simulink subsystem "ElectricMachine1"  (R2022b)
settings: Solver=VariableStepAuto  StartTime=0.0  StopTime=10.0  RelTol=1e-3
undefined symbols (not defined in the file): Spark_MaxTrq_Spd, Spark_Spd_BrkPts
libraries: autolibmappedmotor x1
settings Model: ModifiedByFormat=The MathWorks, Inc.  Creator=The MathWorks, Inc.  LastModifiedBy=The MathWorks, Inc.
settings SolverCC: MaxZcPerStep=1
settings DebuggingCC: UnconnectedInputMsg=warning  UnconnectedOutputMsg=warning  UnconnectedLineMsg=warning
settings ModelReferenceCC: EnableRefExpFcnMdlSchedulingChecks=on
settings RTWCC: DLArmComputeVersion=19.05

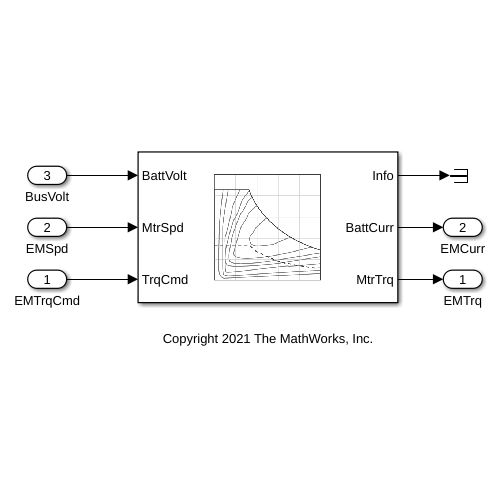
[thumbnail: Simulink's stored preview of the top-level diagram]
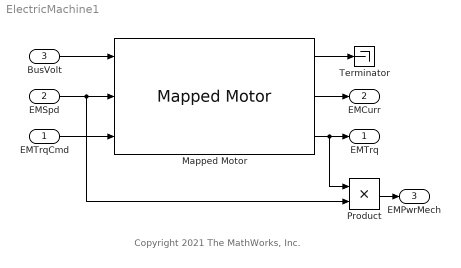
== system ElectricMachine1 ==
  note: Copyright 2021 The MathWorks, Inc.
  EMTrqCmd : Inport
  EMSpd : Inport  Port=2
  BusVolt : Inport  Port=3
  Mapped Motor : autolibmappedmotor/Mapped Motor  port_config=Speed  param_by=Tabulated torque-speed envelope  w_t=Spark_MaxTrq_Spd*(pi/30)  T_t=Spark_MaxTrq  torque_max=0.1  power_max=30  Tc=PlntEM1TimeCnst  param_loss=Tabulated efficiency data  eff=100  w_eff=375  T_eff=0.08  Piron=0  Pbase=0  w_eff_bp=Spark_Spd_BrkPts*(pi/30)  T_eff_bp=Spark_Trq_BrkPts  Temp_eff_bp=Temp_eff_bp  losses_table=losses_table  losses_table_3d=losses_table_3d  efficiency_table=Spark_EffMap  efficiency_table_3d=efficiency_table_3d  J=5e-6  b=1e-5  omega_o=0  T_t_extended=[152.195121951219 157.19263710183 168.578005975641 178.005775209291 192.222891861329 207.776256300937 218.075437684875 229.462130210989 242.676261199004 254.400604378871 265.691686602383 276.934802218937 289.161940741908 307.963362459085 326.3978124807 334.455149023278 343.284814075766 351.285699987009 355.472141711725 355.51814094933 356.300227986961 356.960983702214 357.682405078656 357.728404316261 360 360 360 360 360 360 360 360 360 360 357.728404316261 357.682405078656 356.960983702214 356.300227986961 355.51814094933 355.472141711725 351.285699987009 343.284814075766 334.455149023278 326.3978124807 307.963362459085 289.161940741908 276.934802218937 265.691686602383 254.400604378871 242.676261199004 229.462130210989 218.075437684875 207.776256300937 192.222891861329 178.005775209291 168.578005975641 157.19263710183 152.195121951219]  w_t_extended=[-922.581042604203 -900.589894029074 -858.70199198121 -816.814089933346 -774.926187885482 -733.038285837618 -701.62235930172 -670.206432765822 -638.790506229925 -607.374579694027 -575.958653158129 -544.542726622231 -513.126800086333 -481.710873550435 -450.294947014537 -418.879020478639 -387.463093942741 -356.047167406843 -324.631240870945 -293.215314335047 -261.799387799149 -230.383461263251 -198.967534727354 -167.551608191456 -136.135681655558 -104.71975511966 -73.3038285837618 -31.4159265358979 -0.10471975511966 0.10471975511966 31.4159265358979 73.3038285837618 104.71975511966 136.135681655558 167.551608191456 198.967534727354 230.383461263251 261.799387799149 293.215314335047 324.631240870945 356.047167406843 387.463093942741 418.879020478639 450.294947014537 481.710873550435 513.126800086333 544.542726622231 575.958653158129 607.374579694027 638.790506229925 670.206432765822 701.62235930172 733.038285837618 774.926187885482 816.814089933346 858.70199198121 900.589894029074 922.581042604203]  KLossIron=0  KLossCopper=0  x_w_eff_vec=[-922.581042604203 -876.451990473992 -830.322938343782 -784.193886213572 -738.064834083362 -691.935781953152 -645.806729822942 -599.677677692732 -553.548625562522 -507.419573432311 -461.290521302101 -415.161469171891 -369.032417041681 -322.903364911471 -276.774312781261 -230.645260651051 -184.516208520841 -138.38715639063 -92.2581042604203 -46.1290521302101 -0.10471975511966 0.10471975511966 46.1290521302101 92.2581042604203 138.38715639063 184.516208520841 230.645260651051 276.774312781261 322.903364911471 369.032417041681 415.161469171891 461.290521302101 507.419573432311 553.548625562522 599.677677692732 645.806729822942 691.935781953152 738.064834083362 784.193886213572 830.322938343782 876.451990473992 922.581042604203]  x_T_eff_vec=[-360 -342 -324 -306 -288 -270 -252 -234 -216 -198 -180 -162 -144 -126 -108 -90 -72 -54 -36 -18 -12 -6 -1 1 6 12 18 36 54 72 90 108 126 144 162 180 198 216 234 252 270 288 306 324 342 360]  x_tmp_eff_vec=[233.15 293.15 373.15]  x_losses_mat=[32880788.3584138 31236748.9404931 29592709.5225724 27948670.1046517 26304630.686731 24660591.2688103 23016551.8508896 21372512.432969 19728473.0150483 18084433.5971276 16440394.1792069 13884.0884772239 10771.7570379734 7749.6807578753 6134.87011769928 4832.56736602201 3866.05389281761 3179.96018940172 4104.96733563218 3163.13500321441 1953.70103139714 2152.68909940981 922.581042604203 461.290521302101 1549.93615157506 1660.64587668756 2657.0334027001 3653.42092871264 2989.16257803761 3653.42092871264 4566.7761608908 5779.04765087272 7265.3257105081 9963.87526012538 12703.9409566599 164403.941792069 180844.335971276 197284.730150483 213725.12432969 230165.518508896 246605.912688103 263046.30686731 279486.701046517 295927.095225724 312367.489404931 328807.883584138;31236748.9404931 29674911.4934684 28113074.0464438 26551236.5994191 24989399.1523945 23427561.7053698 21865724.2583452 20303886.8113205 18742049.3642959 17180211.9172712 15602.771698548 12767.0635996566 9499.60867094391 6924.06386523238 5509.12679726509 4502.70261490867 3461.4306459226 2754.56339863254 2743.67579626641 1949.85948442529 1571.56908636716 1945.00304735324 746.607251144512 403.167915618036 1419.85222456787 1367.26510513943 1735.3749411385 2524.1817325651 2603.06241170775 3281.43625233463 4259.55667370361 5206.12482341551 6515.54409718367 8834.63606397784 11713.7808526849 14198.5222456787 171802.119172712 187420.493642959 203038.868113205 218657.242583452 234275.617053698 249893.991523945 265512.365994191 281130.740464438 296749.114934684 312367.489404931;29592709.5225724 28113074.0464438 26633438.5703152 25153803.0941865 23674167.6180579 22194532.1419293 20714896.6658007 19235261.1896721 17755625.7135434 16275990.2374148 14331.6014015502 11300.4926730691 7631.90445456412 6089.03488118773 4719.73038637518 3767.85198912303 2948.38701296471 2484.39633794683 1907.97611364103 1697.63130823963 1181.39908005961 1660.64587668756 679.355131372185 373.645322254702 1245.48440751567 1056.17077757329 1524.47291479918 1793.49754682257 2353.96553020462 2809.81282335536 3586.99509364513 4483.74386705642 5754.13796272241 7173.99018729027 10424.7044909062 13077.5862789146 162759.902374148 177556.257135434 192352.611896721 207148.966658007 221945.321419293 236741.676180579 251538.030941865 266334.385703152 281130.740464438 295927.095225724;27948670.1046517 26551236.5994191 25153803.0941865 23756369.588954 22358936.0837214 20961502.5784888 19564069.0732562 18166635.5680236 16769202.062791 15356.412145413 11858.5416939614 8831.61670783839 6572.29161778993 5200.44366646895 4176.8816017 3325.63899389002 2598.66760619727 2181.88961400748 1643.07290444748 1396.03746776482 930.691645176546 1485.84104756256 616.152339167807 345.045309933972 1129.23919614754 846.929397110658 1270.39409566599 1552.70389470287 2074.97702292111 2484.3262315246 3175.98523916496 3980.5681664201 4940.4214831455 6210.81557881148 8257.56162182891 10939.5047126793 13974.3350523259 167692.02062791 181666.355680236 195640.690732562 209615.025784888 223589.360837214 237563.69588954 251538.030941865 265512.365994191 279486.701046517;26304630.686731 24989399.1523945 23674167.6180579 22358936.0837214 21043704.5493848 19728473.0150483 18413241.4807117 17098009.9463752 15767.011400638 13575.55317773 9616.60883014783 6958.89700707169 5593.75453200021 4382.01843900802 3581.58107573995 2767.74312781261 2214.19450225009 1790.79053786997 1398.43863300005 1155.23191421744 875.94507781322 1360.35479223208 534.460741922435 309.987230315012 1040.67141605754 797.110020810031 1062.81336108004 1328.51670135005 1713.78654474156 2125.62672216008 2657.03340270011 3427.57308948313 4184.82760925266 5314.0668054002 6576.15767168275 8967.48773411285 12421.631157623 14347.9803745806 170980.099463752 184132.414807117 197284.730150483 210437.045493848 223589.360837214 236741.676180579 249893.991523945 263046.30686731;24660591.2688103 23427561.7053698 22194532.1419293 20961502.5784888 19728473.0150483 18495443.4516078 17262413.8881672 ...(+28609 chars)]  x_losses_mat_3d=cat(3,[2 2 2 2 2 2 2 2 2 2 2 2 2 2 2 2 2 2 2 2 2;2 2 2 2 2 2 2 2 2 2 2 2 2 2 2 2 2 2 2 2 2;2 2 2 2 2 2 2 2 2 2 2 2 2 2 2 2 2 2 2 2 2;2 2 2 2 2 2 2 2 2 2 2 2 2 2 2 2 2 2 2 2 2;2 2 2 2 2 2 2 2 2 2 2 2 2 2 2 2 2 2 2 2 2;2 2 2 2 2 2 2 2 2 2 2 2 2 2 2 2 2 2 2 2 2;2 2 2 2 2 2 2 2 2 2 2 2 2 2 2 2 2 2 2 2 2;2 2 2 2 2 2 2 2 2 2 2 2 2 2 2 2 2 2 2 2 2;2 2 2 2 2 2 2 2 2 2 2 2 2 2 2 2 2 2 2 2 2;2 2 2 2 2 2 2 2 2 2 2 2 2 2 2 2 2 2 2 2 2;2 2 2 2 2 2 2 2 2 2 2 2 2 2 2 2 2 2 2 2 2;2 2 2 2 2 2 2 2 2 2 2 2 2 2 2 2 2 2 2 2 2;2 2 2 2 2 2 2 2 2 2 2 2 2 2 2 2 2 2 2 2 2;2 2 2 2 2 2 2 2 2 2 2 2 2 2 2 2 2 2 2 2 2;2 2 2 2 2 2 2 2 2 2 2 2 2 2 2 2 2 2 2 2 2;2 2 2 2 2 2 2 2 2 2 2 2 2 2 2 2 2 2 2 2 2;2 2 2 2 2 2 2 2 2 2 2 2 2 2 2 2 2 2 2 2 2;2 2 2 2 2 2 2 2 2 2 2 2 2 2 2 2 2 2 2 2 2;2 2 2 2 2 2 2 2 2 2 2 2 2 2 2 2 2 2 2 2 2;2 2 2 2 2 2 2 2 2 2 2 2 2 2 2 2 2 2 2 2 2;2 2 2 2 2 2 2 2 2 2 2 2 2 2 2 2 2 2 2 2 2;2 2 2 2 2 2 2 2 2 2 2 2 2 2 2 2 2 2 2 2 2;2 2 2 2 2 2 2 2 2 2 2 2 2 2 2 2 2 2 2 2 2;2 2 2 2 2 2 2 2 2 2 2 2 2 2 2 2 2 2 2 2 2;2 2 2 2 2 2 2 2 2 2 2 2 2 2 2 2 2 2 2 2 2;2 2 2 2 2 2 2 2 2 2 2 2 2 2 2 2 2 2 2 2 2;2 2 2 2 2 2 2 2 2 2 2 2 2 2 2 2 2 2 2 2 2],[1.5 1.5 1.5 1.5 1.5 1.5 1.5 1.5 1.5 1.5 1.5 1.5 1.5 1.5 1.5 1.5 1.5 1.5 1.5 1.5 1.5;1.5 1.5 1.5 1.5 1.5 1.5 1.5 1.5 1.5 1.5 1.5 1.5 1.5 1.5 1.5 1.5 1.5 1.5 1.5 1.5 1.5;1.5 1.5 1.5 1.5 1.5 1.5 1.5 1.5 1.5 1.5 1.5 1.5 1.5 1.5 1.5 1.5 1.5 1.5 1.5 1.5 1.5;1.5 1.5 1.5 1.5 1.5 1.5 1.5 1.5 1.5 1.5 1.5 1.5 1.5 1.5 1.5 1.5 1.5 1.5 1.5 1.5 1.5;1.5 1.5 1.5 1.5 1.5 1.5 1.5 1.5 1.5 1.5 1.5 1.5 1.5 1.5 1.5 1.5 1.5 1.5 1.5 1.5 1.5;1.5 1.5 1.5 1.5 1.5 1.5 1.5 1.5 1.5 1.5 1.5 1.5 1.5 1.5 1.5 1.5 1.5 1.5 1.5 1.5 1.5;1.5 1.5 1.5 1.5 1.5 1.5 1.5 1.5 1.5 1.5 1.5 1.5 1.5 1.5 1.5 1.5 1.5 1.5 1.5 1.5 1.5;1.5 1.5 1.5 1.5 1.5 1.5 1.5 1.5 1.5 1.5 1.5 1.5 1.5 1.5 1.5 1.5 1.5 1.5 1.5 1.5 1.5;1.5 1.5 1.5 1.5 1.5 1.5 1.5 1.5 1.5 1.5 1.5 1.5 1.5 1.5 1.5 1.5 1.5 1.5 1.5 1.5 1.5;1.5 1.5 1.5 1.5 1.5 1.5 1.5 1.5 1.5 1.5 1.5 1.5 1.5 1.5 1.5 1.5 1.5 1.5 1.5 1.5 1.5;1.5 1.5 1.5 1.5 1.5 1.5 1.5 1.5 1.5 1.5 1.5 1.5 1.5 1.5 1.5 1.5 1.5 1.5 1.5 1.5 1.5;1.5 1.5 1.5 1.5 1.5 1.5 1.5 1.5 1.5 1.5 1.5 1.5 1.5 1.5 1.5 1.5 1.5 1.5 1.5 1.5 1.5;1.5 1.5 1.5 1.5 1.5 1.5 1.5 1.5 1.5 1.5 1.5 1.5 1.5 1.5 1.5 1.5 1.5 1.5 1.5 1.5 1.5;1.5 1.5 1.5 1.5 1.5 1.5 1.5 1.5 1.5 1.5 1.5 1.5 1.5 1.5 1.5 1.5 1.5 1.5 1.5 1.5 1.5;1.5 1.5 1.5 1.5 1.5 1.5 1.5 1.5 1.5 1.5 1.5 1.5 1.5 1.5 1.5 1.5 1.5 1.5 1.5 1.5 1.5;1.5 1.5 1.5 1.5 1.5 1.5 1.5 1.5 1.5 1.5 1.5 1.5 1.5 1.5 1.5 1.5 1.5 1.5 1.5 1.5 1.5;1.5 1.5 1.5 1.5 1.5 1.5 1.5 1.5 1.5 1.5 1.5 1.5 1.5 1.5 1.5 1.5 1.5 1.5 1.5 1.5 1.5;1.5 1.5 1.5 1.5 1.5 1.5 1.5 1.5 1.5 1.5 1.5 1.5 1.5 1.5 1.5 1.5 1.5 1.5 1.5 1.5 1.5;1.5 1.5 1.5 1.5 1.5 1.5 1.5 1.5 1.5 1.5 1.5 1.5 1.5 1.5 1.5 1.5 1.5 1.5 1.5 1.5 1.5;1.5 1.5 1.5 1.5 1.5 1.5 1.5 1.5 1.5 1.5 1.5 1.5 1.5 1.5 1.5 1.5 1.5 1.5 1.5 1.5 1.5;1.5 1.5 1.5 1.5 1.5 1.5 1.5 1.5 1.5 1.5 1.5 1.5 1.5 1.5 1.5 1.5 1.5 1.5 1.5 1.5 1.5;1.5 1.5 1.5 1.5 1.5 1.5 1.5 1.5 1.5 1.5 1.5 1.5 1.5 1.5 1.5 1.5 1.5 1.5 1.5 1.5 1.5;1.5 1.5 1.5 1.5 1.5 1.5 1.5 1.5 1.5 1.5 1.5 1.5 1.5 1.5 1.5 1.5 1.5 1.5 1.5 1.5 1.5;1.5 1.5 1.5 1.5 1.5 1.5 1.5 1.5 1.5 1.5 1.5 1.5 1.5 1.5 1.5 1.5 1.5 1.5 1.5 1.5 1.5;1.5 1.5 1.5 1.5 1.5 1.5 1.5 1.5 1.5 1.5 1.5 1.5 1.5 1.5 1.5 1.5 1.5 1.5 1.5 1.5 1.5;1.5 1.5 1.5 1.5 1.5 1.5 1.5 1.5 1.5 1.5 1.5 1.5 1.5 1.5 1.5 1.5 1.5 1.5 1.5 1.5 1.5;1.5 1.5 1.5 1.5 1.5 1.5 1.5 1.5 1.5 1.5 1.5 1.5 1.5 1.5 1.5 1.5 1.5 1.5 1.5 1.5 1.5],[1.9 1.9 1.9 1.9 1.9 1.9 1.9 1.9 1.9 1.9 1.9 1.9 1.9 1.9 1.9 1.9 1.9 1.9 1.9 1.9 1.9;1.9 1.9 1.9 1.9 1.9 1.9 1.9 1.9 1.9 1.9 1.9 1.9 1.9 1.9 1.9 1.9 1.9 1.9 1.9 1.9 1.9;1.9 1.9 1.9 1.9 1.9 1.9 1.9 1.9 1.9 1.9 1.9 1.9 1.9 1.9 1.9 1.9 1.9 1.9 1.9 1.9 1.9;1.9 1.9 1.9 1.9 1.9 1.9 1.9 1.9 1.9 1.9 1.9 1.9 1.9 1.9 1.9 1.9 1.9 1.9 1.9 1.9 1.9;1.9 1.9 1.9 1.9 1.9 1.9 1.9 1.9 1.9 1.9 1.9 1.9 1.9 1.9 1.9 1.9 1.9 1.9 1.9 1.9 1.9;1.9 1.9 1.9 1.9 1.9 1.9 1.9 1.9 1.9 1.9 1.9 1.9 1.9 1.9 1.9 1.9 1.9 1.9 1.9 1.9 1.9;1.9 1.9 1.9 1.9 1.9 1.9 1.9 1.9 1.9 1.9 1.9 1.9 1.9 1.9 1.9 1.9 1.9 1.9 1.9 1.9 1.9 ...(+1680 chars)])  CalLossMapData={'BaseCageProjectFileName','';'BaseMbcProjectFileName','';'TaskName','Calibrate Motor Loss Map';'ChildTasks',{{'DataName','';'TaskName','Import Loss Data'},{'TaskName','Generate Response Models'},{'TaskName','Generate Calibration'},{'TaskName','Update Block Parameters'}}}  CalLossWithTempMapData={}  aMode=6  RefBlkName='autolibmappedmotor/Mapped Motor'
  Product : Product
  Terminator : Terminator
  EMTrq : Outport  VectorParamsAs1DForOutWhenUnconnected=off
  EMCurr : Outport  Port=2  VectorParamsAs1DForOutWhenUnconnected=off
  EMPwrMech : Outport  Port=3
  wires:
  EMSpd/1 -> Product/2, Mapped Motor/2
  EMTrqCmd/1 -> Mapped Motor/3
  BusVolt/1 -> Mapped Motor/1
  Mapped Motor/1 -> Terminator/1
  Mapped Motor/2 -> EMCurr/1
  Mapped Motor/3 -> EMTrq/1, Product/1
  Product/1 -> EMPwrMech/1
